simulink model "ds1_plant"  (R2019a)
settings: Solver=ode14x  StartTime=0  StopTime=.1660  FixedStep=.00001  RelTol=1e-3  EnableMultiTasking=on
model workspace (MAT data in the model file):
  Ankle_L_D = 0.125126243033
  Ankle_L_S = 0.0328154604487
  Ankle_R_D = 0.245807097642
  Ankle_R_S = 0.682954357178
  BeginTimePlantModel = 1.52
  F_C = 0.0618
  F_H = 0.107
  F_I = 0.0103200285075
  F_L = 0.2471
  F_M = 1.2499
  F_W = 0.11
  GRF_HD = 941.037069119
  GRF_HS = 1691.11560066
  GRF_VD = 12300.8672242
  GRF_VS = 71710.3574634
  HAT_I = 5.06800535295
  HAT_L = 0.549
  HAT_M = 58.9182
  HAT_a = 0.2
  HAT_b = 0.13
  Hip_L_D = 0.0332143791481
  Hip_L_S = 0.0516603438036
  Hip_R_D = 0.145088103411
  Hip_R_S = 0.15911410017
  Knee_L_D = 0.0558982452805
  Knee_L_S = 0.00250387295429
  Knee_R_D = 0.0619293882143
  Knee_R_S = 0.0623339259595
  M.stance_ankle = [1765.48010254; 1788.2947998; 1801.50634766; 1802.40429688; 1790.12036133; 1765.5970459; 1729.50976562; 1674.8092041; 1600.0246582; 1501.14147949; 1381.22302246; 1242.12426758; 1082.7635498; 907.980651855; 727.113342285; 543.440551758; 362.143432617; 226.103546143; 114.855056763; 32.033405304; -22.7033824921]
  M.strike_ankle = [12.0487298965; 10.9718074799; 8.85982036591; 5.59524440765; 1.13871026039; -13.008562088; -43.4141731262; -71.6242828369; -90.0088500977; -129.552642822; -144.145645142; -134.347595215; -123.832756042; -128.809188843; -124.52722168; -129.464447021; -133.513626099; -129.856002808; -27.7111053467; -24.4621429443; -21.4752922058]
  M.stance_knee = [-629.495910645; -596.171386719; -568.967468262; -540.194824219; -501.200286865; -447.069915771; -401.211364746; -346.565490723; -304.740966797; -268.297088623; -226.840194702; -203.759414673; -185.193283081; -154.514907837; -116.670310974; -68.1001358032; 42.0167694092; 89.6592941284; 156.330490112; 190.886077881; 195.93536377]
  M.strike_knee = [-320.084838867; -285.409179688; -247.132583618; -206.970336914; -166.625717163; -127.234100342; -367.266143799; -389.615447998; -193.257507324; -28.3099937439; 100.478012085; 66.7882461548; 23.6458110809; 98.8639831543; 196.848922729; 275.537872314; 325.650054932; 345.530578613; 31.0123653412; 27.6135787964; 23.9695453644]
  M.stance_hip = [-726.74621582; -776.746520996; -796.444030762; -799.321777344; -803.850097656; -820.8515625; -806.054992676; -788.789978027; -730.75994873; -646.090698242; -564.684631348; -446.737030029; -329.32800293; -250.149597168; -211.835510254; -217.825714111; -367.795379639; -417.873718262; -518.579711914; -564.6328125; -557.363220215]
  M.strike_hip = [468.511047363; 404.565124512; 338.414215088; 273.085113525; 211.394561768; 168.620697021; 788.185791016; 947.539489746; 618.310302734; 409.466156006; 219.211090088; 314.827087402; 429.747497559; 303.987304688; 111.515075684; -16.5758476257; -87.0600891113; -121.653160095; 25.2755432129; 33.0600204468; 40.5797348022]
  S_I = 0.0584148214017
  S_L = 0.447
  S_M = 4.0083
  S_R1 = 0.06
  S_R2 = 0.08
  T_I = 0.243990929891
  T_L = 0.476
  T_M = 8.62
  T_R1 = 0.08
  T_R2 = 0.1
  bodymass = 86.2
  p_stance_ankle = 14.9539905036
  p_stance_hip = -24.9413676415
  p_stance_knee = -2.50807459996
  p_swing_ankle = 4.11757124464
  p_swing_hip = 18.3000604838
  p_swing_knee = -3.41741510381
  polyfit_stance_ankle = [-863347.977095 222377.922877 -7468.35453889 -9.40558010807 -153.06789694]
  polyfit_stance_hip = [-279786636.688 114363391.625 -15725654.0525 856134.662579 -22930.0516399 481.110496147 63.2694363354]
  polyfit_stance_knee = [-122862314.114 52903969.6705 -7988612.27678 487806.049871 -8969.32141641 330.337585729 -54.0526736443]
  polyfit_swing_ankle = [49510154320.8 -30205907167.6 7312588550.85 -888915044.437 56385922.5861 -1769074.37171 25613.4020917 -113.306543933 -1.03720591697]
  polyfit_swing_hip = [538683495113 -366532634246 101719653645 -14750073882.9 1184454520.37 -50949861.1242 1019832.60417 -6310.84925925 -38.0907282261]
  polyfit_swing_knee = [352478408737 -233011269241 62650744932.5 -8775138187.04 678489689.503 -28060179.8998 545151.783137 -3282.03325692 -26.455631467]
  stance_hip_D = -0.1
  stance_hip_I = 0
  stance_hip_P = -1
  swing_hip_D = -0.1
  swing_hip_I = 0
  swing_hip_P = -1
  u_stance_ankle = [-149.998419046 -149.999798728 -149.999934988 -149.999961517 -149.999969736 -149.999974943]
  u_stance_knee = [27.5743588885 23.6652812799 -29.6745015743 17.5659545156 14.7975024083 14.5439260216]
  u_swing_ankle = [-7.72010188045 6.45863736131 5.78565475448 4.91572634254 7.49750636005 7.99781009736]
  u_swing_knee = [-14.9490992242 -14.9954340728 -14.9993338993 -14.9998188648 -14.9999159851 -14.9999404756]
  w_stance_ankle = 4.93716584662
  w_stance_hip = 2.61448296759
  w_stance_knee = 13.9723172709
  w_swing_ankle = -56.5478745686
  w_swing_hip = 73.7662715002
  w_swing_knee = 18.6992302324
  x_planar_p = 0
  x_planar_v = 0
  y_planar_p = 0
  y_planar_v = 0
  yout = [8.16988597066 8.1627557225 8.15559878707 8.14841513681 8.14120474348 8.13396757813 8.12670361115 8.11941281227 8.1120951506 8.10475059463 8.09737911226 8.08998067083 ... (8000 elements, 1000x8)]
  z_planar_p = -10.3139246991
  z_planar_w = -47.4942945829
undefined symbols (not defined in the file or in its folder): X, Y, Z
libraries: nesl_utility x87, sm_lib x50, fl_lib x24, fl_ps_legacy_lib x16, simulink x4
(part 1 of 4)
settings Model: OrderedModelArguments=off  Creator=6438sunj  LastModifiedBy=8842thayerj
settings DataIOCC: LimitDataPoints=on  SaveFormat=Array  SignalLoggingSaveFormat=ModelDataLogs  ReturnWorkspaceOutputs=off  SignalLoggingName=SPE_DataLog  OutputOption=SpecifiedOutputTimes  OutputTimes=spe_config.time
settings OptimizationCC: ExpressionDepthLimit=2147483647  LifeSpan=inf
settings DebuggingCC: UnderspecifiedInitializationDetection=Classic  MergeDetectMultiDrivingBlocksExec=none  SolverPrmCheckMsg=warning  StateNameClashWarn=warning  SFUnexpectedBacktrackingDiag=warning  SFNoUnconditionalDefaultTransitionDiag=warning  SFExecutionAtInitializationDiag=none  ArithmeticOperatorsInVariantConditions=warning
settings HardwareCC: ProdBitPerPointer=32  ProdBitPerSizeT=32  ProdBitPerPtrDiffT=32  ProdLargestAtomicFloat=None  ProdIntDivRoundTo=Undefined  ProdEndianess=Unspecified  ProdWordSize=32  ProdHWDeviceType=32-bit Generic
settings ModelReferenceCC: PropagateSignalLabelsOutOfModel=off
settings SFSimCC: SimUseLocalCustomCode=off
settings RTWCC: RTWUseLocalCustomCode=off
settings CodeAppCC: StateflowObjectComments=on
settings GRTTargetCC: TargetLangStandard=C89/C90 (ANSI)  GeneratePreprocessorConditionals=Disable all
settings ConfigComp: CovMetricSettings=dw  CovHtmlReporting=on  CovSaveCumulativeToWorkspaceVar=on  CovSaveSingleToWorkspaceVar=on  CovExternalEMLEnable=off
settings SimscapeCC: SimscapeNormalizeSystem=off
settings ConfigurationSet: Description=SimMechanics 2G
settings DiagnosticsConfigSet: SimMechanicsUnconnectedFramePorts=none
settings ExplorerConfigSet: InternalSimMechanicsExplorerSettings="<ExplorerConfiguration><canonicalview>default</canonicalview><TilePanel><TileInfo><Tiles Columns=\"1\" Count=\"1\" Rows=\"1\"><Column Left=\"2\" Weight=\"1\"/><Column Left=\"715\"/><Row Top=\"2\" Weight=\"1\"/><Row Top=\"555\"/><Tile Height=\"1\" Width=\"1\" X=\"0\" Y=\"0\"/></Tiles></TileInfo><SceneInfo><SceneViewer><BGColor><R>0.60000002384185791</R><G>0.60000002384185791</G><B>0.60000002384185791</B></BGColor><Camera><Position><X>2.3238188926266905</X><Y>0.29801581507321606</Y><Z>0.5830879823253462</Z></Position><Center><X>0</X><Y>0.29801581507321606</Y><Z>0.5830879823253462</Z></Center><Up><X>-0</X><Y>0</Y><Z>1</Z></Up><Left>-0.37797235250473021</Left><Right>0.37797235250473021</Right><Bottom>-0.82692947387695315</Bottom><Top>0.82692947387695315</Top></Camera></SceneViewer></SceneInfo></TilePanel></ExplorerConfiguration>"

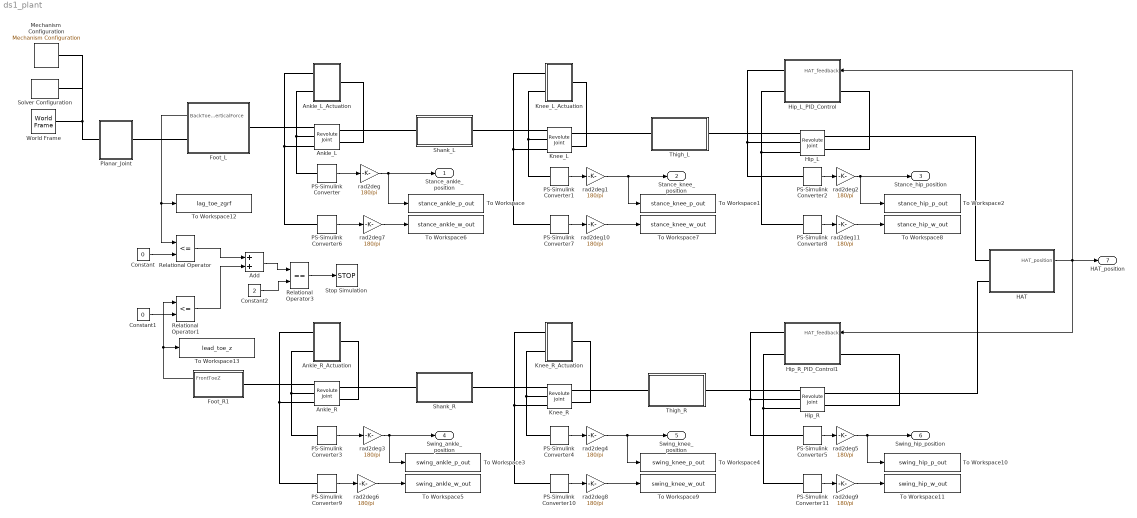
== system ds1_plant ==
  Add : Sum  OutMin=0  OutMax=2
  Ankle_L : sm_lib/Joints/Revolute Joint  SenseConstraintForce=off  SenseConstraintForceX=off  SenseConstraintForceY=off  SenseConstraintForceZ=off  SenseConstraintTorque=off  SenseConstraintTorqueX=off  SenseConstraintTorqueY=off  SenseConstraintTorqueZ=off  SenseTotalForce=off  SenseTotalForceX=off  SenseTotalForceY=off  SenseTotalForceZ=off  SenseTotalTorque=off  SenseTotalTorqueX=off  SenseTotalTorqueY=off  SenseTotalTorqueZ=off  CompositeWrenchDir=FollowerOnBase  CompositeWrenchFrame=BaseFrame  EquilibriumPosition=0  EquilibriumPositionUnits=deg  SpringStiffness=Ankle_L_S  SpringStiffnessUnits=N*m/deg  DampingCoefficient=Ankle_L_D  DampingCoefficientUnits=N*m/(deg/s)  TorqueActuationMode=InputTorque  MotionActuationMode=ComputedMotion  SensePosition=on  SenseVelocity=on  SenseAcceleration=off  SenseTorqueForce=off  SenseLowerLimitTorqueForce=off  SenseUpperLimitTorqueForce=off  LowerLimitSpecify=off  LowerLimitBound=-90  LowerLimitBoundUnits=deg  LowerLimitStiffness=1e4  LowerLimitStiffnessUnits=N*m/deg  LowerLimitDamping=10  LowerLimitDampingUnits=N*m/(deg/s)  LowerLimitTransitionRegionWidth=0.1  LowerLimitTransitionRegionWidthUnits=deg  UpperLimitSpecify=off  UpperLimitBound=90  UpperLimitBoundUnits=deg  UpperLimitStiffness=1e4  UpperLimitStiffnessUnits=N*m/deg  UpperLimitDamping=10  UpperLimitDampingUnits=N*m/(deg/s)  UpperLimitTransitionRegionWidth=0.1  UpperLimitTransitionRegionWidthUnits=deg  PositionTargetSpecify=on  PositionTargetPriority=High  PositionTargetValue=p_stance_ankle  PositionTargetValueUnits=deg  VelocityTargetSpecify=on  VelocityTargetPriority=High  VelocityTargetValue=w_stance_ankle  VelocityTargetValueUnits=deg/s
  Ankle_L_Actuation : Subsystem
  Ankle_R : sm_lib/Joints/Revolute Joint  SenseConstraintForce=off  SenseConstraintForceX=off  SenseConstraintForceY=off  SenseConstraintForceZ=off  SenseConstraintTorque=off  SenseConstraintTorqueX=off  SenseConstraintTorqueY=off  SenseConstraintTorqueZ=off  SenseTotalForce=off  SenseTotalForceX=off  SenseTotalForceY=off  SenseTotalForceZ=off  SenseTotalTorque=off  SenseTotalTorqueX=off  SenseTotalTorqueY=off  SenseTotalTorqueZ=off  CompositeWrenchDir=FollowerOnBase  CompositeWrenchFrame=BaseFrame  EquilibriumPosition=0  EquilibriumPositionUnits=deg  SpringStiffness=Ankle_R_S  SpringStiffnessUnits=N*m/deg  DampingCoefficient=Ankle_R_D  DampingCoefficientUnits=N*m/(deg/s)  TorqueActuationMode=InputTorque  MotionActuationMode=ComputedMotion  SensePosition=on  SenseVelocity=on  SenseAcceleration=off  SenseTorqueForce=off  SenseLowerLimitTorqueForce=off  SenseUpperLimitTorqueForce=off  LowerLimitSpecify=off  LowerLimitBound=-90  LowerLimitBoundUnits=deg  LowerLimitStiffness=1e4  LowerLimitStiffnessUnits=N*m/deg  LowerLimitDamping=10  LowerLimitDampingUnits=N*m/(deg/s)  LowerLimitTransitionRegionWidth=0.1  LowerLimitTransitionRegionWidthUnits=deg  UpperLimitSpecify=off  UpperLimitBound=90  UpperLimitBoundUnits=deg  UpperLimitStiffness=1e4  UpperLimitStiffnessUnits=N*m/deg  UpperLimitDamping=10  UpperLimitDampingUnits=N*m/(deg/s)  UpperLimitTransitionRegionWidth=0.1  UpperLimitTransitionRegionWidthUnits=deg  PositionTargetSpecify=on  PositionTargetPriority=High  PositionTargetValue=p_swing_ankle  PositionTargetValueUnits=deg  VelocityTargetSpecify=on  VelocityTargetPriority=High  VelocityTargetValue=w_swing_ankle  VelocityTargetValueUnits=deg/s
  Ankle_R_Actuation : Subsystem
  Constant : Constant  Value=0
  Constant1 : Constant  Value=0
  Constant2 : Constant  Value=2
  Foot_L : Subsystem  mask{F_L=F_L, F_H=F_H, F_C=F_C, F_W=F_W, F_M=F_M, F_I=F_I}
      mask prompts: F_L "Foot Length (m)"; F_H "Foot Height (m)"; F_C "Heel to Mid Foot (m)"; F_W "Foot Width (m)"; F_M "Foot Mass (kg)"; F_I "Foot Moment of Inertia (kg*m^2)"
      mask init:
      | % Defines the cross section of the thigh
      | 
      | F_cross_section = [(F_L-F_C),0;0, F_H; -F_C,0 ];
  Foot_R1 : Subsystem  mask{F_L=F_L, F_H=F_H, F_C=F_C, F_W=F_W, F_M=F_M, F_I=F_I}
      mask prompts: F_L "Foot Length (m)"; F_H "Foot Height (m)"; F_C "Heel to Mid Foot (m)"; F_W "Foot Width (m)"; F_M "Foot Mass (kg)"; F_I "Foot Moment of Inertia (kg*m^2)"
      mask init:
      | % Defines the cross section of the thigh
      | 
      | F_cross_section = [(F_L-F_C),0;0, F_H; -F_C,0; ];
  HAT : Subsystem  mask{HAT_a=HAT_a, HAT_b=HAT_b, HAT_L=HAT_L, HAT_M=HAT_M, HAT_I=HAT_I}
      mask prompts: HAT_a "Long Axis Length (m)"; HAT_b "Short Axis Length (m)"; HAT_L "HAT Height (m)"; HAT_M "Mass (kg)"; HAT_I "Moment of Inertia (kg*m^2)"
      mask init:
      | % Defines the cross-section of the HAT
      | theta = ([0:.01:360]*(pi/180))';
      | HAT_cross_section = [HAT_a*cos(theta), HAT_b*sin(theta)];
  Hip_L : sm_lib/Joints/Revolute Joint  SenseConstraintForce=off  SenseConstraintForceX=off  SenseConstraintForceY=off  SenseConstraintForceZ=off  SenseConstraintTorque=off  SenseConstraintTorqueX=off  SenseConstraintTorqueY=off  SenseConstraintTorqueZ=off  SenseTotalForce=off  SenseTotalForceX=off  SenseTotalForceY=off  SenseTotalForceZ=off  SenseTotalTorque=off  SenseTotalTorqueX=off  SenseTotalTorqueY=off  SenseTotalTorqueZ=off  CompositeWrenchDir=FollowerOnBase  CompositeWrenchFrame=BaseFrame  EquilibriumPosition=0  EquilibriumPositionUnits=deg  SpringStiffness=Hip_L_S  SpringStiffnessUnits=N*m/deg  DampingCoefficient=Hip_L_D  DampingCoefficientUnits=N*m/(deg/s)  TorqueActuationMode=InputTorque  MotionActuationMode=ComputedMotion  SensePosition=on  SenseVelocity=on  SenseAcceleration=off  SenseTorqueForce=off  SenseLowerLimitTorqueForce=off  SenseUpperLimitTorqueForce=off  LowerLimitSpecify=off  LowerLimitBound=-90  LowerLimitBoundUnits=deg  LowerLimitStiffness=1e4  LowerLimitStiffnessUnits=N*m/deg  LowerLimitDamping=10  LowerLimitDampingUnits=N*m/(deg/s)  LowerLimitTransitionRegionWidth=0.1  LowerLimitTransitionRegionWidthUnits=deg  UpperLimitSpecify=off  UpperLimitBound=90  UpperLimitBoundUnits=deg  UpperLimitStiffness=1e4  UpperLimitStiffnessUnits=N*m/deg  UpperLimitDamping=10  UpperLimitDampingUnits=N*m/(deg/s)  UpperLimitTransitionRegionWidth=0.1  UpperLimitTransitionRegionWidthUnits=deg  PositionTargetSpecify=on  PositionTargetPriority=High  PositionTargetValue=p_stance_hip  PositionTargetValueUnits=deg  VelocityTargetSpecify=on  VelocityTargetPriority=High  VelocityTargetValue=w_stance_hip  VelocityTargetValueUnits=deg/s
  Hip_L_PID_Control : Subsystem
  Hip_R : sm_lib/Joints/Revolute Joint  SenseConstraintForce=off  SenseConstraintForceX=off  SenseConstraintForceY=off  SenseConstraintForceZ=off  SenseConstraintTorque=off  SenseConstraintTorqueX=off  SenseConstraintTorqueY=off  SenseConstraintTorqueZ=off  SenseTotalForce=off  SenseTotalForceX=off  SenseTotalForceY=off  SenseTotalForceZ=off  SenseTotalTorque=off  SenseTotalTorqueX=off  SenseTotalTorqueY=off  SenseTotalTorqueZ=off  CompositeWrenchDir=FollowerOnBase  CompositeWrenchFrame=BaseFrame  EquilibriumPosition=0  EquilibriumPositionUnits=deg  SpringStiffness=Hip_R_S  SpringStiffnessUnits=N*m/deg  DampingCoefficient=Hip_R_D  DampingCoefficientUnits=N*m/(deg/s)  TorqueActuationMode=InputTorque  MotionActuationMode=ComputedMotion  SensePosition=on  SenseVelocity=on  SenseAcceleration=off  SenseTorqueForce=off  SenseLowerLimitTorqueForce=off  SenseUpperLimitTorqueForce=off  LowerLimitSpecify=off  LowerLimitBound=-90  LowerLimitBoundUnits=deg  LowerLimitStiffness=1e4  LowerLimitStiffnessUnits=N*m/deg  LowerLimitDamping=10  LowerLimitDampingUnits=N*m/(deg/s)  LowerLimitTransitionRegionWidth=0.1  LowerLimitTransitionRegionWidthUnits=deg  UpperLimitSpecify=off  UpperLimitBound=90  UpperLimitBoundUnits=deg  UpperLimitStiffness=1e4  UpperLimitStiffnessUnits=N*m/deg  UpperLimitDamping=10  UpperLimitDampingUnits=N*m/(deg/s)  UpperLimitTransitionRegionWidth=0.1  UpperLimitTransitionRegionWidthUnits=deg  PositionTargetSpecify=on  PositionTargetPriority=High  PositionTargetValue=p_swing_hip  PositionTargetValueUnits=deg  VelocityTargetSpecify=on  VelocityTargetPriority=High  VelocityTargetValue=w_swing_hip  VelocityTargetValueUnits=deg/s
  Hip_R_PID_Control1 : Subsystem
  Knee_L : sm_lib/Joints/Revolute Joint  SenseConstraintForce=off  SenseConstraintForceX=off  SenseConstraintForceY=off  SenseConstraintForceZ=off  SenseConstraintTorque=off  SenseConstraintTorqueX=off  SenseConstraintTorqueY=off  SenseConstraintTorqueZ=off  SenseTotalForce=off  SenseTotalForceX=off  SenseTotalForceY=off  SenseTotalForceZ=off  SenseTotalTorque=off  SenseTotalTorqueX=off  SenseTotalTorqueY=off  SenseTotalTorqueZ=off  CompositeWrenchDir=FollowerOnBase  CompositeWrenchFrame=BaseFrame  EquilibriumPosition=0  EquilibriumPositionUnits=deg  SpringStiffness=Knee_L_S  SpringStiffnessUnits=N*m/deg  DampingCoefficient=Knee_L_D  DampingCoefficientUnits=N*m/(deg/s)  TorqueActuationMode=InputTorque  MotionActuationMode=ComputedMotion  SensePosition=on  SenseVelocity=on  SenseAcceleration=off  SenseTorqueForce=off  SenseLowerLimitTorqueForce=off  SenseUpperLimitTorqueForce=off  LowerLimitSpecify=off  LowerLimitBound=-90  LowerLimitBoundUnits=deg  LowerLimitStiffness=1e4  LowerLimitStiffnessUnits=N*m/deg  LowerLimitDamping=10  LowerLimitDampingUnits=N*m/(deg/s)  LowerLimitTransitionRegionWidth=0.1  LowerLimitTransitionRegionWidthUnits=deg  UpperLimitSpecify=off  UpperLimitBound=90  UpperLimitBoundUnits=deg  UpperLimitStiffness=1e4  UpperLimitStiffnessUnits=N*m/deg  UpperLimitDamping=10  UpperLimitDampingUnits=N*m/(deg/s)  UpperLimitTransitionRegionWidth=0.1  UpperLimitTransitionRegionWidthUnits=deg  PositionTargetSpecify=on  PositionTargetPriority=High  PositionTargetValue=p_stance_knee  PositionTargetValueUnits=deg  VelocityTargetSpecify=on  VelocityTargetPriority=High  VelocityTargetValue=w_stance_knee  VelocityTargetValueUnits=deg/s
  Knee_L_Actuation : Subsystem
  Knee_R : sm_lib/Joints/Revolute Joint  SenseConstraintForce=off  SenseConstraintForceX=off  SenseConstraintForceY=off  SenseConstraintForceZ=off  SenseConstraintTorque=off  SenseConstraintTorqueX=off  SenseConstraintTorqueY=off  SenseConstraintTorqueZ=off  SenseTotalForce=off  SenseTotalForceX=off  SenseTotalForceY=off  SenseTotalForceZ=off  SenseTotalTorque=off  SenseTotalTorqueX=off  SenseTotalTorqueY=off  SenseTotalTorqueZ=off  CompositeWrenchDir=FollowerOnBase  CompositeWrenchFrame=BaseFrame  EquilibriumPosition=0  EquilibriumPositionUnits=deg  SpringStiffness=Knee_R_S  SpringStiffnessUnits=N*m/deg  DampingCoefficient=Knee_R_D  DampingCoefficientUnits=N*m/(deg/s)  TorqueActuationMode=InputTorque  MotionActuationMode=ComputedMotion  SensePosition=on  SenseVelocity=on  SenseAcceleration=off  SenseTorqueForce=off  SenseLowerLimitTorqueForce=off  SenseUpperLimitTorqueForce=off  LowerLimitSpecify=off  LowerLimitBound=-90  LowerLimitBoundUnits=deg  LowerLimitStiffness=1e4  LowerLimitStiffnessUnits=N*m/deg  LowerLimitDamping=10  LowerLimitDampingUnits=N*m/(deg/s)  LowerLimitTransitionRegionWidth=0.1  LowerLimitTransitionRegionWidthUnits=deg  UpperLimitSpecify=off  UpperLimitBound=90  UpperLimitBoundUnits=deg  UpperLimitStiffness=1e4  UpperLimitStiffnessUnits=N*m/deg  UpperLimitDamping=10  UpperLimitDampingUnits=N*m/(deg/s)  UpperLimitTransitionRegionWidth=0.1  UpperLimitTransitionRegionWidthUnits=deg  PositionTargetSpecify=on  PositionTargetPriority=High  PositionTargetValue=p_swing_knee  PositionTargetValueUnits=deg  VelocityTargetSpecify=on  VelocityTargetPriority=High  VelocityTargetValue=w_swing_knee  VelocityTargetValueUnits=deg/s
  Knee_R_Actuation : Subsystem
  Mechanism  Configuration : sm_lib/Utilities/Mechanism Configuration  UniformGravity=Constant  GravityVector=[0 0 -9.81]  GravityUnits=m/s^2  LinearizationDelta=0.001
  PS-Simulink Converter{,1..11} (12 alike) : nesl_utility/PS-Simulink Converter  PhysicalDomain=network_engine_domain  SubClassName=ps_output  LeftPortType=input  RightPortType=output  PseudoPeriodic=off  Frequencies=[]  Unit=1  AffineConversion=off
  Planar_Joint : Subsystem
  Relational Operator : RelationalOperator  Operator=<=  OutDataTypeStr=fixdt('boolean', 'DataTypeOverride', 'Off')  RndMeth=Simplest
  Relational Operator1 : RelationalOperator  Operator=<=  OutDataTypeStr=fixdt('boolean', 'DataTypeOverride', 'Off')  RndMeth=Simplest
  Relational Operator3 : RelationalOperator  Operator===  OutDataTypeStr=fixdt('boolean', 'DataTypeOverride', 'Off')  RndMeth=Simplest
  Shank_L : Subsystem  mask{S_R2=S_R2, S_R1=S_R1, S_L=S_L, S_M=S_M, S_I=S_I}
      mask prompts: S_R2 "Proximal End Radius (m)"; S_R1 "Distal End Radius (m)"; S_L "Shank Length (m)"; S_M "Shank Mass (kg)"; S_I "Shank Moment of Inertia (kg*m^2)"
      mask init:
      | % Defines the cross section of the thigh
      | 
      | S_cross_section = [0,0; S_R1, 0; S_R2, S_L; 0,S_L];
  Shank_R : Subsystem  mask{S_R2=S_R2, S_R1=S_R1, S_L=S_L, S_M=S_M, S_I=S_I}
      mask prompts: S_R2 "Proximal End Radius (m)"; S_R1 "Distal End Radius (m)"; S_L "Shank Length (m)"; S_M "Shank Mass (kg)"; S_I "Shank Moment of Inertia (kg*m^2)"
      mask init:
      | % Defines the cross section of the thigh
      | 
      | S_cross_section = [0,0; S_R1, 0; S_R2, S_L; 0,S_L];
  Solver Configuration : nesl_utility/Solver Configuration  PhysicalDomain=network_engine_domain  SubClassName=solver  LeftPortType=input  RightPortType=generic  Tones=[]  Harmonics=[]  SimulateNoise=off  Profile=off  UseLocalSampling=off  EnableSwitchedLinearOptims=on  FrequencyDomain=off  UseCCode=off  RelTol=0.001  AbsTol=1e-06  MinStep=1e-09  ToWorkspace=off  RevertToSquareIcSolve=off  NumHomotopyIterations=100  PhasorMode=off  PhasorModeNumHarmonics=1  DoDC=off  ResidualTolerance=1e-9  UseLocalSolver=off  LocalSolverChoice=NE_BACKWARD_EULER_ADVANCER  LocalSolverSampleTime=.001  DoFixedCost=off  MaxNonlinIter=3  MaxModeIter=2  LinearAlgebra=Sparse  EquationFormulation=NE_TIME_EF  DelaysMemoryBudget=1024  AutomaticFiltering=on  FilteringTimeConstant=0.001  PartitionStorageMethod=AS_NEEDED  PartitionMemoryBudget=1024  PartitionMethod=FAST
  Stop Simulation : Stop
  Thigh_L : Subsystem  mask{T_R2=T_R2, T_R1=T_R1, T_L=T_L, T_M=T_M, T_I=T_I}
      mask prompts: T_R2 "Proximal End Radius (m)"; T_R1 "Distal End Radius (m)"; T_L "Thigh Length (m)"; T_M "Thigh Mass (kg)"; T_I "Thigh Moment of Inertia (kg*m^2)"
      mask init:
      | % Defines the cross section of the thigh
      | 
      | T_cross_section = [0,0; T_R1, 0; T_R2, T_L; 0,T_L];
  Thigh_R : Subsystem  mask{T_R2=T_R2, T_R1=T_R1, T_L=T_L, T_M=T_M, T_I=T_I}
      mask prompts: T_R2 "Proximal End Radius (m)"; T_R1 "Distal End Radius (m)"; T_L "Thigh Length (m)"; T_M "Thigh Mass (kg)"; T_I "Thigh Moment of Inertia (kg*m^2)"
      mask init:
      | % Defines the cross section of the thigh
      | 
      | T_cross_section = [0,0; T_R1, 0; T_R2, T_L; 0,T_L];
  To Workspace : ToWorkspace  VariableName=stance_ankle_p_out  SampleTime=-1
  To Workspace1 : ToWorkspace  VariableName=stance_knee_p_out  SampleTime=-1
  To Workspace10 : ToWorkspace  VariableName=swing_hip_p_out  SampleTime=-1
  To Workspace11 : ToWorkspace  VariableName=swing_hip_w_out  SampleTime=-1
  To Workspace12 : ToWorkspace  VariableName=lag_toe_zgrf  SampleTime=-1
  To Workspace13 : ToWorkspace  VariableName=lead_toe_z  SampleTime=-1
  To Workspace2 : ToWorkspace  VariableName=stance_hip_p_out  SampleTime=-1
  To Workspace3 : ToWorkspace  VariableName=swing_ankle_p_out  SampleTime=-1
  To Workspace4 : ToWorkspace  VariableName=swing_knee_p_out  SampleTime=-1
  To Workspace5 : ToWorkspace  VariableName=swing_ankle_w_out  SampleTime=-1
  To Workspace6 : ToWorkspace  VariableName=stance_ankle_w_out  SampleTime=-1
  To Workspace7 : ToWorkspace  VariableName=stance_knee_w_out  SampleTime=-1
  To Workspace8 : ToWorkspace  VariableName=stance_hip_w_out  SampleTime=-1
  To Workspace9 : ToWorkspace  VariableName=swing_knee_w_out  SampleTime=-1
  World Frame : sm_lib/Frames and Transforms/World Frame
  rad2deg{,1..11} (12 alike) : Gain  Gain=180/pi
  Stance_ankle_position : Outport
  Stance_knee_position : Outport  Port=2
  Stance_hip_position : Outport  Port=3
  Swing_ankle_position : Outport  Port=4
  Swing_knee_position : Outport  Port=5
  Swing_hip_position : Outport  Port=6
  HAT_position : Outport  Port=7
  wires:
  PS-Simulink Converter/1 -> rad2deg/1
  PS-Simulink Converter1/1 -> rad2deg1/1
  PS-Simulink Converter2/1 -> rad2deg2/1
  PS-Simulink Converter3/1 -> rad2deg3/1
  PS-Simulink Converter4/1 -> rad2deg4/1
  PS-Simulink Converter5/1 -> rad2deg5/1
  rad2deg/1 -> To Workspace/1, Stance_ankle_position/1
  rad2deg1/1 -> Stance_knee_position/1, To Workspace1/1
  rad2deg2/1 -> To Workspace2/1, Stance_hip_position/1
  rad2deg3/1 -> To Workspace3/1, Swing_ankle_position/1
  rad2deg4/1 -> To Workspace4/1, Swing_knee_position/1
  rad2deg5/1 -> To Workspace10/1, Swing_hip_position/1
  HAT/1(HAT_position) -> HAT_position/1, Hip_L_PID_Control/1(HAT_feedback), Hip_R_PID_Control1/1(HAT_feedback)
  PS-Simulink Converter6/1 -> rad2deg7/1
  rad2deg7/1 -> To Workspace6/1
  PS-Simulink Converter7/1 -> rad2deg10/1
  rad2deg10/1 -> To Workspace7/1
  PS-Simulink Converter8/1 -> rad2deg11/1
  rad2deg11/1 -> To Workspace8/1
  PS-Simulink Converter11/1 -> rad2deg9/1
  rad2deg9/1 -> To Workspace11/1
  PS-Simulink Converter10/1 -> rad2deg8/1
  rad2deg8/1 -> To Workspace9/1
  PS-Simulink Converter9/1 -> rad2deg6/1
  rad2deg6/1 -> To Workspace5/1
  Constant2/1 -> Relational Operator3/2
  Add/1 -> Relational Operator3/1
  Relational Operator1/1 -> Add/2
  Relational Operator/1 -> Add/1
  Relational Operator3/1 -> Stop Simulation/1
  Constant1/1 -> Relational Operator1/2
  Foot_R1/1(FrontToeZ) -> To Workspace13/1, Relational Operator1/1
  Constant/1 -> Relational Operator/2
  Foot_L/1(BackToeVerticalForce) -> To Workspace12/1, Relational Operator/1
  connections:
  World Frame/RConn1 -- Planar_Joint/LConn1 -- Mechanism  Configuration/RConn1 -- Solver Configuration/RConn1
  Planar_Joint/RConn1 -- Foot_L/RConn1
  Foot_L/LConn1 -- Ankle_L/RConn1
  Ankle_L/LConn1 -- Shank_L/RConn1
  Knee_L/RConn1 -- Shank_L/LConn1
  Knee_L/LConn1 -- Thigh_L/RConn1
  Hip_L/RConn1 -- Thigh_L/LConn1
  Hip_L/LConn1 -- HAT/LConn1
  Foot_R1/LConn1 -- Ankle_R/RConn1
  Ankle_R/LConn1 -- Shank_R/RConn1
  Knee_R/RConn1 -- Shank_R/LConn1
  Knee_R/LConn1 -- Thigh_R/RConn1
  Hip_R/RConn1 -- Thigh_R/LConn1
  Hip_R/LConn1 -- HAT/LConn2
  Ankle_L_Actuation/LConn1 -- Ankle_L/LConn2
  Ankle_R/LConn2 -- Ankle_R_Actuation/LConn1
  Knee_L_Actuation/LConn1 -- Knee_L/LConn2
  Knee_R_Actuation/LConn1 -- Knee_R/LConn2
  Ankle_L/RConn3 -- PS-Simulink Converter6/LConn1 -- Ankle_L_Actuation/RConn1
  Ankle_R/RConn3 -- PS-Simulink Converter9/LConn1 -- Ankle_R_Actuation/RConn1
  Knee_L/RConn3 -- PS-Simulink Converter7/LConn1 -- Knee_L_Actuation/RConn1
  Knee_R/RConn3 -- PS-Simulink Converter10/LConn1 -- Knee_R_Actuation/RConn1
  Hip_R/RConn3 -- PS-Simulink Converter11/LConn1 -- Hip_R_PID_Control1/RConn2
  Ankle_L/RConn2 -- Ankle_L_Actuation/RConn2 -- PS-Simulink Converter/LConn1
  Knee_L/RConn2 -- PS-Simulink Converter1/LConn1 -- Knee_L_Actuation/RConn2
  Hip_L/RConn2 -- PS-Simulink Converter2/LConn1 -- Hip_L_PID_Control/RConn1
  Ankle_R/RConn2 -- PS-Simulink Converter3/LConn1 -- Ankle_R_Actuation/RConn2
  Knee_R/RConn2 -- PS-Simulink Converter4/LConn1 -- Knee_R_Actuation/RConn2
  Hip_R/RConn2 -- PS-Simulink Converter5/LConn1 -- Hip_R_PID_Control1/RConn1
  Hip_L/RConn3 -- PS-Simulink Converter8/LConn1 -- Hip_L_PID_Control/RConn2
  Hip_L_PID_Control/LConn1 -- Hip_L/LConn2
  Hip_R_PID_Control1/LConn1 -- Hip_R/LConn2
